simulink model "Copy_of_E5ABC_"  (R2021a)
settings: Solver=FixedStepAuto  StartTime=0.0  StopTime=0.08  FixedStep=1e-7  MaxStep=1e-7  RelTol=1e-6
libraries: spsSeriesRLCBranchLib x38, spsDiodeLib x27, spsCurrentMeasurementLib x18, spsGroundLib x12, simulink x12, spsParallelRLCBranchLib x12, spsVoltageMeasurementLib x11, spsThyristorLib x9, spsMosfetLib x6, spsDCVoltageSourceLib x6, spsIdealSwitchLib x6, spsControlledVoltageSourceLib x6
(part 2 of 2)

== system Copy_of_E5ABC_/Gate Drive/Pulse Trafo #5/Subsystem ==
  D2 : spsDiodeLib/Diode  Ron=0.001  Lon=0  Vf=0.7  IC=0  UseSnubber=off  Rs=inf  Cs=0  Measurements=off
  Data Type Conversion1 : DataTypeConversion  OutDataTypeStr=boolean
  R (for simulation) : spsSeriesRLCBranchLib/Series RLC Branch  LConnTagsString=__new0  RConnTagsString=__new0  BranchType=R  Resistance=100000  Inductance=60e-3  SetiL0=off  InitialCurrent=0  Capacitance=1e-6  Setx0=off  InitialVoltage=0  Measurements=None
  Relay1 : Relay  OnSwitchValue=0.36  OffSwitchValue=0.2
  Rg : spsSeriesRLCBranchLib/Series RLC Branch  LConnTagsString=__new0  RConnTagsString=__new0  BranchType=R  Resistance=20  Inductance=60e-3  SetiL0=off  InitialCurrent=0  Capacitance=1e-6  Setx0=off  InitialVoltage=0  Measurements=None
  Rgk : spsSeriesRLCBranchLib/Series RLC Branch  LConnTagsString=__new0  RConnTagsString=__new0  BranchType=R  Resistance=10  Inductance=60e-3  SetiL0=off  InitialCurrent=0  Capacitance=1e-6  Setx0=off  InitialVoltage=0  Measurements=None
  V_gk : spsVoltageMeasurementLib/Voltage Measurement  PhasorSimulation=off  OutputType=Complex  PSBequivalent=0
  +ve : PMIOPort  Side=Left
  -ve : PMIOPort  Port=2  Side=Left
  O : Outport
  wires:
  Relay1/1 -> Data Type Conversion1/1
  Data Type Conversion1/1 -> O/1
  V_gk/1 -> Relay1/1
  connections:
  V_gk/LConn2 -- Rgk/LConn1 -- R (for simulation)/LConn1 -- -ve/RConn1
  +ve/RConn1 -- Rg/RConn1
  Rg/LConn1 -- D2/LConn1 -- R (for simulation)/RConn1
  Rgk/RConn1 -- V_gk/LConn1 -- D2/RConn1

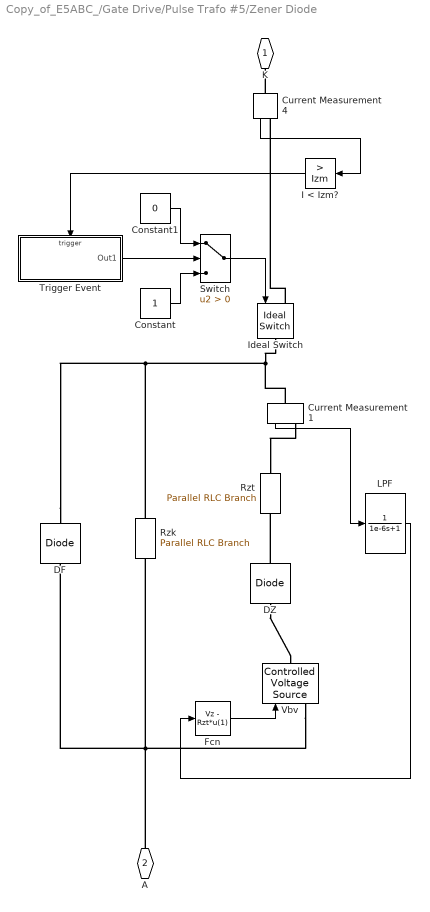
== system Copy_of_E5ABC_/Gate Drive/Pulse Trafo #5/Zener Diode ==
  Constant : Constant
  Constant1 : Constant  Value=0
  Current Measurement1 : spsCurrentMeasurementLib/Current Measurement  PhasorSimulation=off  OutputType=Complex  PSBequivalent=0
  Current Measurement4 : spsCurrentMeasurementLib/Current Measurement  PhasorSimulation=off  OutputType=Complex  PSBequivalent=0
  DF : spsDiodeLib/Diode  Ron=Ron  Lon=0  Vf=Vf  IC=0  UseSnubber=off  Rs=1000  Cs=0  Measurements=off
      settings: AttributesFormatString=\n
  DZ : spsDiodeLib/Diode  Ron=1e-6  Lon=0  Vf=0  IC=0  UseSnubber=off  Rs=100  Cs=inf  Measurements=off
      settings: AttributesFormatString=\n
  Fcn : Fcn  Expr=Vz - Rzt*u(1)
  I < Izm? : simulink/Logic and Bit Operations/Compare To Constant  relop=>  const=Izm  OutDataTypeStr=boolean
  Ideal Switch : spsIdealSwitchLib/Ideal Switch  Ron=0.001  Lon=0  IC=1  Rs=1e5  Cs=0  Measurements=off
  LPF : TransferFcn  Denominator=[1e-6 1]
  Rzk : spsParallelRLCBranchLib/Parallel RLC Branch  LConnTagsString=a  RConnTagsString=__new0  BranchType=R  Resistance=Rzk  Inductance=1.0  SetiL0=off  InitialCurrent=0  Capacitance=1e-5  Setx0=off  InitialVoltage=0  Measurements=None
  Rzt : spsParallelRLCBranchLib/Parallel RLC Branch  LConnTagsString=a  RConnTagsString=__new0  BranchType=R  Resistance=Rzt  Inductance=1.0  SetiL0=off  InitialCurrent=0  Capacitance=1e-5  Setx0=off  InitialVoltage=0  Measurements=None
  Switch : Switch  Criteria=u2 > Threshold
  Trigger Event : Subsystem  TreatAsAtomicUnit=on
  Vbv : spsControlledVoltageSourceLib/Controlled Voltage Source  Initialize=off  Source_Type=DC  Amplitude=0  Phase=0  Frequency=0  Measurements=None
  K : PMIOPort  Side=Left
  A : PMIOPort  Port=2  Side=Right
  wires:
  Constant1/1 -> Switch/1
  Constant/1 -> Switch/3
  Trigger Event/1(Out1) -> Switch/2
  Switch/1 -> Ideal Switch/1
  I < Izm?/1 -> Trigger Event/Trigger
  LPF/1 -> Fcn/1
  Current Measurement1/1 -> LPF/1
  Current Measurement4/1 -> I < Izm?/1
  Fcn/1 -> Vbv/1
  connections:
  Vbv/LConn1 -- Rzk/LConn1 -- DF/LConn1 -- A/RConn1
  Ideal Switch/LConn1 -- Current Measurement4/RConn1
  DF/RConn1 -- Ideal Switch/RConn1 -- Current Measurement1/LConn1 -- Rzk/RConn1
  Current Measurement1/RConn1 -- Rzt/RConn1
  DZ/LConn1 -- Rzt/LConn1
  Current Measurement4/LConn1 -- K/RConn1
  DZ/RConn1 -- Vbv/RConn1

== system Copy_of_E5ABC_/Gate Drive/Pulse Trafo #6/Subsystem ==
  D2 : spsDiodeLib/Diode  Ron=0.001  Lon=0  Vf=0.7  IC=0  UseSnubber=off  Rs=inf  Cs=0  Measurements=off
  Data Type Conversion1 : DataTypeConversion  OutDataTypeStr=boolean
  R (for simulation) : spsSeriesRLCBranchLib/Series RLC Branch  LConnTagsString=__new0  RConnTagsString=__new0  BranchType=R  Resistance=100000  Inductance=60e-3  SetiL0=off  InitialCurrent=0  Capacitance=1e-6  Setx0=off  InitialVoltage=0  Measurements=None
  Relay1 : Relay  OnSwitchValue=0.36  OffSwitchValue=0.2
  Rg : spsSeriesRLCBranchLib/Series RLC Branch  LConnTagsString=__new0  RConnTagsString=__new0  BranchType=R  Resistance=20  Inductance=60e-3  SetiL0=off  InitialCurrent=0  Capacitance=1e-6  Setx0=off  InitialVoltage=0  Measurements=None
  Rgk : spsSeriesRLCBranchLib/Series RLC Branch  LConnTagsString=__new0  RConnTagsString=__new0  BranchType=R  Resistance=10  Inductance=60e-3  SetiL0=off  InitialCurrent=0  Capacitance=1e-6  Setx0=off  InitialVoltage=0  Measurements=None
  V_gk : spsVoltageMeasurementLib/Voltage Measurement  PhasorSimulation=off  OutputType=Complex  PSBequivalent=0
  +ve : PMIOPort  Side=Left
  -ve : PMIOPort  Port=2  Side=Left
  O : Outport
  wires:
  V_gk/1 -> Relay1/1
  Data Type Conversion1/1 -> O/1
  Relay1/1 -> Data Type Conversion1/1
  connections:
  D2/RConn1 -- V_gk/LConn1 -- Rgk/RConn1
  R (for simulation)/RConn1 -- D2/LConn1 -- Rg/LConn1
  +ve/RConn1 -- Rg/RConn1
  -ve/RConn1 -- R (for simulation)/LConn1 -- Rgk/LConn1 -- V_gk/LConn2

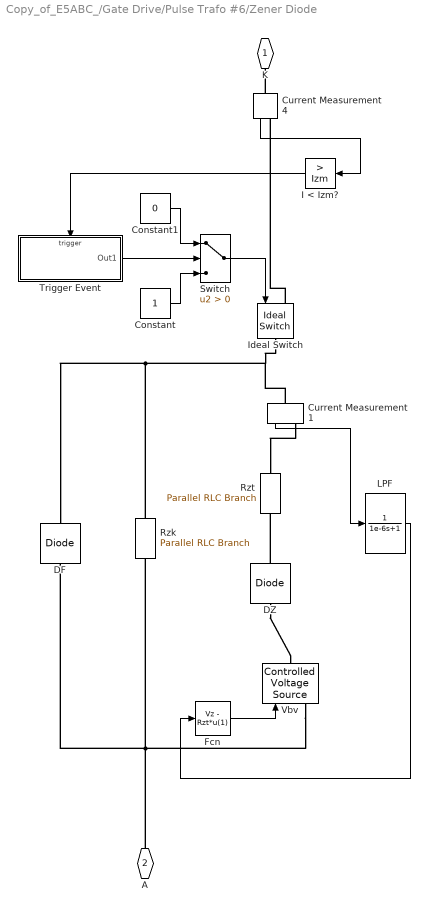
== system Copy_of_E5ABC_/Gate Drive/Pulse Trafo #6/Zener Diode ==
  Constant : Constant
  Constant1 : Constant  Value=0
  Current Measurement1 : spsCurrentMeasurementLib/Current Measurement  PhasorSimulation=off  OutputType=Complex  PSBequivalent=0
  Current Measurement4 : spsCurrentMeasurementLib/Current Measurement  PhasorSimulation=off  OutputType=Complex  PSBequivalent=0
  DF : spsDiodeLib/Diode  Ron=Ron  Lon=0  Vf=Vf  IC=0  UseSnubber=off  Rs=1000  Cs=0  Measurements=off
      settings: AttributesFormatString=\n
  DZ : spsDiodeLib/Diode  Ron=1e-6  Lon=0  Vf=0  IC=0  UseSnubber=off  Rs=100  Cs=inf  Measurements=off
      settings: AttributesFormatString=\n
  Fcn : Fcn  Expr=Vz - Rzt*u(1)
  I < Izm? : simulink/Logic and Bit Operations/Compare To Constant  relop=>  const=Izm  OutDataTypeStr=boolean
  Ideal Switch : spsIdealSwitchLib/Ideal Switch  Ron=0.001  Lon=0  IC=1  Rs=1e5  Cs=0  Measurements=off
  LPF : TransferFcn  Denominator=[1e-6 1]
  Rzk : spsParallelRLCBranchLib/Parallel RLC Branch  LConnTagsString=a  RConnTagsString=__new0  BranchType=R  Resistance=Rzk  Inductance=1.0  SetiL0=off  InitialCurrent=0  Capacitance=1e-5  Setx0=off  InitialVoltage=0  Measurements=None
  Rzt : spsParallelRLCBranchLib/Parallel RLC Branch  LConnTagsString=a  RConnTagsString=__new0  BranchType=R  Resistance=Rzt  Inductance=1.0  SetiL0=off  InitialCurrent=0  Capacitance=1e-5  Setx0=off  InitialVoltage=0  Measurements=None
  Switch : Switch  Criteria=u2 > Threshold
  Trigger Event : Subsystem  TreatAsAtomicUnit=on
  Vbv : spsControlledVoltageSourceLib/Controlled Voltage Source  Initialize=off  Source_Type=DC  Amplitude=0  Phase=0  Frequency=0  Measurements=None
  K : PMIOPort  Side=Left
  A : PMIOPort  Port=2  Side=Right
  wires:
  Fcn/1 -> Vbv/1
  Current Measurement4/1 -> I < Izm?/1
  Current Measurement1/1 -> LPF/1
  LPF/1 -> Fcn/1
  I < Izm?/1 -> Trigger Event/Trigger
  Switch/1 -> Ideal Switch/1
  Trigger Event/1(Out1) -> Switch/2
  Constant/1 -> Switch/3
  Constant1/1 -> Switch/1
  connections:
  DZ/RConn1 -- Vbv/RConn1
  Current Measurement4/LConn1 -- K/RConn1
  DZ/LConn1 -- Rzt/LConn1
  Current Measurement1/RConn1 -- Rzt/RConn1
  Rzk/RConn1 -- Current Measurement1/LConn1 -- Ideal Switch/RConn1 -- DF/RConn1
  Ideal Switch/LConn1 -- Current Measurement4/RConn1
  A/RConn1 -- DF/LConn1 -- Rzk/LConn1 -- Vbv/LConn1

== system Copy_of_E5ABC_/Gate Drive/Pulse Trafo #1/Zener Diode/Trigger Event ==
  Trigger : TriggerPort  VariantControl=Variant  ShowOutputPort=on
  Out1 : Outport
  wires:
  Trigger/1 -> Out1/1

== system Copy_of_E5ABC_/Gate Drive/Pulse Trafo #2/Zener Diode/Trigger Event ==
  Trigger : TriggerPort  VariantControl=Variant  ShowOutputPort=on
  Out1 : Outport
  wires:
  Trigger/1 -> Out1/1

== system Copy_of_E5ABC_/Gate Drive/Pulse Trafo #3/Zener Diode/Trigger Event ==
  Trigger : TriggerPort  VariantControl=Variant  ShowOutputPort=on
  Out1 : Outport
  wires:
  Trigger/1 -> Out1/1

== system Copy_of_E5ABC_/Gate Drive/Pulse Trafo #4/Zener Diode/Trigger Event ==
  Trigger : TriggerPort  VariantControl=Variant  ShowOutputPort=on
  Out1 : Outport
  wires:
  Trigger/1 -> Out1/1

== system Copy_of_E5ABC_/Gate Drive/Pulse Trafo #5/Zener Diode/Trigger Event ==
  Trigger : TriggerPort  VariantControl=Variant  ShowOutputPort=on
  Out1 : Outport
  wires:
  Trigger/1 -> Out1/1

== system Copy_of_E5ABC_/Gate Drive/Pulse Trafo #6/Zener Diode/Trigger Event ==
  Trigger : TriggerPort  VariantControl=Variant  ShowOutputPort=on
  Out1 : Outport
  wires:
  Trigger/1 -> Out1/1
